simulink model "Model_LQR"  (R2018a)
settings: Solver=VariableStepAuto  StartTime=0.0  StopTime=10.0  RelTol=1e-3
values from neighbouring files (symbols this model uses):
  pulse = 4    [CEE_10.m]    (also in CEE_10_performance.m; CEE_10_unc.m; CEE_9.m; CEE_9_performance.m)
  x0 = [50,0,10,0,0]'*pi/180    [CEE_10.m]    (also in CEE_10_performance.m; CEE_11.m; CEE_9.m; CEE_9_performance.m)
undefined symbols (not defined in the file or in its folder): A, B, C, K
settings Model: Creator=miguelsilva  LastModifiedBy=leonardopedroso
settings DebuggingCC: LibraryContextMissingDiagnostic=warning
settings SFSimCC: SimUseLocalCustomCode=on
settings RTWCC: RTWUseLocalCustomCode=on

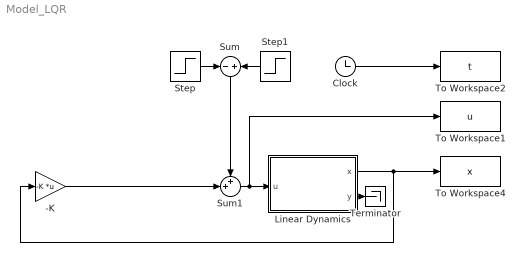
== system Model_LQR ==
  -K : Gain  Gain=-K  Multiplication=Matrix(K*u) (u vector)
  Clock : Clock
  Linear Dynamics : Subsystem
  Step : Step  Time=5.1  After=pulse  SampleTime=0
  Step1 : Step  Time=5  After=pulse  SampleTime=0
  Sum : Sum  Inputs=-|+
  Sum1 : Sum  Inputs=++|
  Terminator : Terminator
  To Workspace1 : ToWorkspace  VariableName=u  SampleTime=-1
  To Workspace2 : ToWorkspace  VariableName=t  SampleTime=-1
  To Workspace4 : ToWorkspace  VariableName=x  SampleTime=-1
  wires:
  Clock/1 -> To Workspace2/1
  Linear Dynamics/1(x) -> -K/1, To Workspace4/1
  Step/1 -> Sum/1
  Step1/1 -> Sum/2
  Sum/1 -> Sum1/1
  -K/1 -> Sum1/2
  Sum1/1 -> To Workspace1/1, Linear Dynamics/1(u)
  Linear Dynamics/2(y) -> Terminator/1

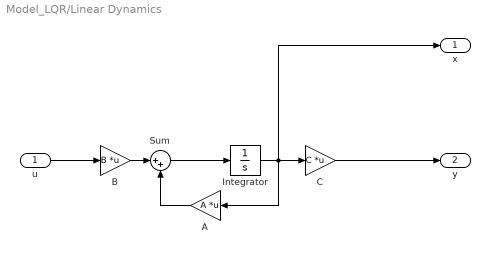
== system Model_LQR/Linear Dynamics ==
  u : Inport
  A : Gain  Gain=A  Multiplication=Matrix(K*u) (u vector)
  B : Gain  Gain=B  Multiplication=Matrix(K*u) (u vector)
  C : Gain  Gain=C  Multiplication=Matrix(K*u) (u vector)
  Integrator : Integrator  InitialCondition=x0
  Sum : Sum  Inputs=|++
  x : Outport
  y : Outport  Port=2
  wires:
  u/1 -> B/1
  C/1 -> y/1
  B/1 -> Sum/1
  Sum/1 -> Integrator/1
  A/1 -> Sum/2
  Integrator/1 -> x/1, C/1, A/1
